simulink model "machanical_model"  (Simulink 7.0)
settings: Solver=ode45  StartTime=0.0  StopTime=4.0  RelTol=1e-3
undefined symbols (not defined in the file or in its folder): z0
settings Model: Creator=sergei  LastModifiedBy=Sergei Gusev

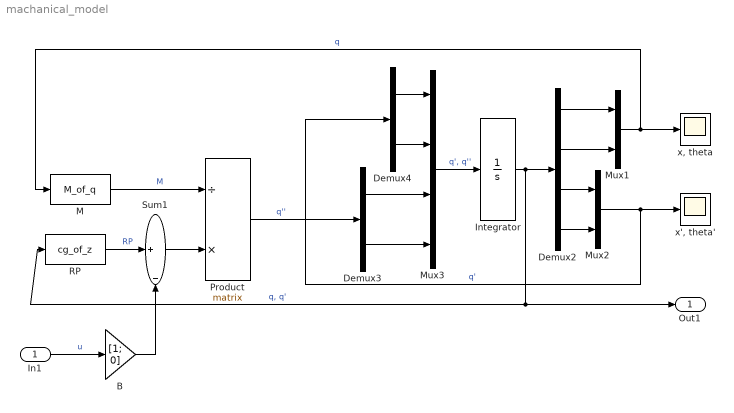
== system machanical_model ==
  In1 : Inport  OutDataType=sfix(16)  OutScaling=2^0
  B : Gain  Gain=[1; 0]  ParameterDataType=sfix(16)  ParameterScaling=2^0  OutDataType=sfix(16)  OutScaling=2^0
  Demux2 : Demux
  Demux3 : Demux  Outputs=2
  Demux4 : Demux  Outputs=2
  Integrator : Integrator  InitialCondition=z0  ZeroCross=off
  M : MATLABFcn  MATLABFcn=M_of_q  OutputDimensions=[2 2]  OutputSignalType=real  Output1D=off
  Mux1 : Mux  Inputs=2
  Mux2 : Mux  Inputs=2
  Mux3 : Mux
  Product : Product  Inputs=/*  Multiplication=Matrix(*)  OutDataType=sfix(16)  OutScaling=2^0  RndMeth=Zero
  RP : MATLABFcn  MATLABFcn=cg_of_z  OutputDimensions=[2 1]  OutputSignalType=real  Output1D=off
  Sum1 : Sum  Inputs=|+-  OutDataType=sfix(16)  OutScaling=2^0
  "x', theta'" : Scope
      settings: Tag=phi  YMin=-1.1  YMax=0.3  SaveName=ScopeData2
  "x, theta" : Scope
      settings: Tag=theta  YMin=-1.1  YMax=0.3
  Out1 : Outport  OutDataType=sfix(16)  OutScaling=2^0
  wires:
  Mux3/1 -> Integrator/1  "q', q''"
  Demux3/1 -> Mux3/3
  Demux3/2 -> Mux3/4
  Product/1 -> Demux3/1  "q''"
  M/1 -> Product/1  "M"
  Sum1/1 -> Product/2
  RP/1 -> Sum1/1  "RP"
  Demux4/1 -> Mux3/1
  Demux4/2 -> Mux3/2
  Demux2/3 -> Mux2/1
  Demux2/4 -> Mux2/2
  Mux2/1 -> Demux4/1, "x', theta'"/1  "q'"
  Demux2/2 -> Mux1/2
  Demux2/1 -> Mux1/1
  B/1 -> Sum1/2
  Mux1/1 -> M/1, "x, theta"/1  "q"
  Integrator/1 -> RP/1, Out1/1, Demux2/1  "q, q'"
  In1/1 -> B/1  "u"
